simulink model "filter_test"  (R2013a)
settings: Solver=ode45  StartTime=0.0  StopTime=60  RelTol=1e-3
undefined symbols (not defined in the file or in its folder): fdesignblkfcn, gcbh
settings Model: Creator=dholley  LastModifiedBy=dholley

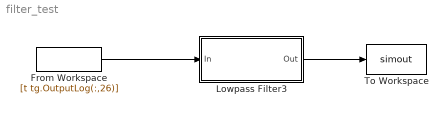
== system filter_test ==
  From Workspace : FromWorkspace  VariableName=[t tg.OutputLog(:,26)]  SampleTime=.001
  Lowpass Filter3 : Subsystem  DialogController=fdesignblkfcn  InitFcn=fdesignblkfcn(gcbh, {'InitFcn'});  mask(Lowpass Filter){}
      mask help: Design a lowpass filter
      settings: CopyFcn=fdesignblkfcn(gcbh, {'CopyFcn'});
      mask Help: helpview(mapfilelocation('dsp'), 'dsplowpassfilter');
      mask Display: disp('Lowpass')
  To Workspace : ToWorkspace  VariableName=simout  SampleTime=.001  SaveFormat=Timeseries
  wires:
  Lowpass Filter3/1(Out) -> To Workspace/1
  From Workspace/1 -> Lowpass Filter3/1(In)

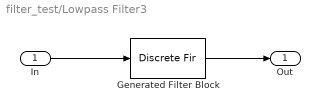
== system filter_test/Lowpass Filter3 ==
  In : Inport
  Generated Filter Block : DiscreteFir  Tag=BlockMethodSubSystem  Coefficients=[0.00089245422298423057 7.4164336383486214e-05 7.6895717906471793e-05 7.908073415934273e-05 8.1181328409573022e-05 8.2612264663942266e-05 8.3861775260315324e-05 8.430522686922199e-05 8.4498978316928462e-05 8.378964444078949e-05 8.2898898551494364e-05 8.1096809270959826e-05 7.9364095360265319e-05 7.6614644333435045e-05 7.4043967667513483e-05 6.7959558569482799e-05 6.3485151437216777e-05 5.8126469094912686e-05 5.1150790278283375e-05 4.3865245212162994e-05 3.534526297379703e-05 2.610117261526209e-05 1.5722825516115016e-05 4.4680397682335046e-06 -7.8443886726743553e-06 -2.1118204296247545e-05 -3.542415256008733e-05 -5.089267652868385e-05 -6.7538946304533014e-05 -8.5623045518801134e-05 -0.00010434332098532004 -0.00012428219350524294 -0.00014590128495966376 -0.00016824750095483865 -0.0001921513429811244 -0.0002170982435519722 -0.00024344535581068789 -0.00027089602516835955 -0.00029967817345930535 -0.00032960072652682437 -0.00036084654838391831 -0.00039330019912986501 -0.00042705837173662728 -0.00046193429050254151 -0.00049790049078254764 -0.00053503906040128842 -0.00057357418822451874 -0.00061283744245703149 -0.00065345238541316677 -0.00069494081212886092 -0.00073751244359737938 -0.00078093026784587351 -0.00082531481424835793 -0.00087047827964123557 -0.00091651137150473394 -0.00096322357724722119 -0.00101064406168457 -0.0010585502930350516 -0.001107022332570773 -0.0011559338066055597 -0.0012053241853571648 -0.0012547524577068321 -0.0013045840271248561 -0.0013543916305556413 -0.0014042302376472018 -0.0014539348569981402 -0.0015034653949292779 -0.0015526598893101239 -0.0016014682404827554 -0.0016496995105394485 -0.0016972886015228844 -0.0017440493871673029 -0.0017899753431801083 -0.0018348638398668143 -0.0018786322865944689 -0.0019210060168792405 -0.0019621065476833903 -0.0020015815079050497 -0.0020393717330077234 -0.0020753757126098669 -0.0021094137815858881 -0.0021413702122777089 -0.0021710925176990025 -0.002198430394740913 -0.0022232547374456189 -0.0022454262409327226 -0.002264842766889901 -0.0022813153587343434 -0.0022947137067009845 -0.0023048827011817223 -0.0023117786638524665 -0.0023151551461553432 -0.0023149084569998655 -0.0023109918088351483 -0.0023031639534982734 -0.0022913803198994992 -0.0022754647056114322 -0.0022553309387236811 -0.0022308486853840634 -0.0022019350394811704 -0.0021684661618028875 -0.002130327767941342 -0.0020874188394236779 -0.0020396789606537047 -0.001987016093022259 -0.0019293170869327469 -0.0018665113880511209 -0.0017986124659580757 -0.0017254225905697675 -0.0016469940700789179 -0.0015632134291013464 -0.0014740767471187635 -0.0013795315731099458 -0.0012795710391340686 -0.0011741460537713383 -0.0010632536105911103 -0.00094688867896254624 -0.00082508391688205737 -0.00069781253412155083 -0.0005651076979314209 -0.00042699540737199107 -0.00028356328801770671 -0.00013474840359720098 1.9291264939995346e-05 0.00017854510295218584 0.0003429253663132626 0.00051234781135882292 0.00068673006353458805 0.00086598290072887739 0.0010499925016817047 0.0012386347223156185 0.0014317843844408313 0.001629335592659237 0.0018311252269483957 0.0020370053837582918 0.002246809138751399 0.0024604275410246928 0.002677615338577505 0.0028982240895013148 0.0031220814093816558 0.0033489553273743189 0.0035786847868045368 0.0038110362237878991 0.0040458046328414061 0.0042827495643627082 0.004521668142147329 0.0047623228749378585 0.0050044650098530494 0.0052478476329321476 0.0054922415104306562 0.0057373964050013325 0.0059830266845192978 0.0062288828817872828 0.0064747396184742928 0.0067202655015642177 0.0069652603633950476 0.007209402244197638 0.0074524466897019827 0.0076940986635125139 0.0079341177633470601 0.0081722013548371636 0.0084080835039177758 0.0086414844798954078 0.0088721587718167058 0.0090998037801884868 0.0093241584088986466 0.0095449505502529022 0.0097619564334823737 0.0099748402455274304 0.010183423059863989 0.010387389377647757 0.010586522484157996 0.010780563419240139 0.010969293521403568 0.011152448282229287 ...(+4955 chars)]  InputProcessing=Columns as channels (frame based)
  Out : Outport
  wires:
  In/1 -> Generated Filter Block/1
  Generated Filter Block/1 -> Out/1
